simulink model "SM_Offshore_Windturbine"  (R2021a)
settings: Solver=ode4  StartTime=0.0  StopTime=par.sym.Ttot  FixedStep=par.sym.max_dt  MaxStep=par.sym.max_dt  RelTol=1e-3
model workspace: external: MATLAB File C:\Users\d053704\Desktop\MOST\Structure\CAD\CAD_DataFile.m (data not in the file)
undefined symbols (not defined in the file): par, smiData, X, Y, Z
libraries: sm_lib x50, simulink_extras x29, vrlib x18, nesl_utility x10, dspstat3 x9, sharedutil x5, eeGeneralControl x2
(part 3 of 4)

== system SM_Offshore_Windturbine/WIND TURBINE/BODIES MOTIONS/Simscape/Nacelle ==
  Nacelle : sm_lib/Body Elements/File Solid  ExtGeomFileName=Nacelle_Default_sldprt.STEP  UnitType=FromFile  ExtGeomFileUnits=m  StepReaderType=HEX  ExportConvexHullGeometry=off  InertiaType=Custom  Mass=smiData.Solid(5).mass  MassUnits=kg  CenterOfMass=smiData.Solid(5).CoM  CenterOfMassUnits=m  MomentsOfInertia=[eps eps eps]  MomentsOfInertiaUnits=kg*m^2  ProductsOfInertia=[0 0 0]  ProductsOfInertiaUnits=kg*m^2  BasedOnType=Density  Density=1000  DensityUnits=kg/m^3  DoExposeReferenceFrame=on  SerializedFrames=<Frames/>  GraphicType=FromGeometry  MarkerShape=Sphere  MarkerSize=10  GraphicVisPropType=SimpleVisualProperties  GraphicDiffuseColor=smiData.Solid(5).color  GraphicSpecularColor=[0.5 0.5 0.5 1.0]  GraphicAmbientColor=[0.15 0.15 0.15 1.0]  GraphicEmissiveColor=[0.0 0.0 0.0 1.0]  GraphicShininess=75  GraphicOpacity=smiData.Solid(5).opacity
  ReferenceFrame : sm_lib/Frames and Transforms/Reference Frame
  Transform1 : sm_lib/Frames and Transforms/Rigid Transform  TranslationMethod=Cartesian  TranslationStandardOffset=0  TranslationLengthUnit=m  TranslationStandardAxis=+Z  TranslationCartesianOffset=smiData.RigidTransform(9).translation  TranslationROffset=0  TranslationROffsetUnits=m  TranslationZOffset=0  TranslationZOffsetUnits=m  TranslationThetaOffset=0  TranslationThetaOffsetUnits=deg  RotationMethod=ArbitraryAxis  RotationAngleUnits=rad  RotationStandardAxis=+Z  RotationAngle=smiData.RigidTransform(9).angle  RotationArbitraryAxis=smiData.RigidTransform(9).axis  FollAlignAxisA=+X  BaseAlignAxisA=+Y  FollAlignAxisB=+Y  BaseAlignAxisB=+Z  RotationSequenceAxes=FollowerAxes  RotationSequence=XYX  RotationSequenceAngles=[0 0 0]  RotationSequenceAnglesUnits=deg  RotationMatrix=[1 0 0; 0 1 0; 0 0 1]
  Transform2 : sm_lib/Frames and Transforms/Rigid Transform  TranslationMethod=Cartesian  TranslationStandardOffset=0  TranslationLengthUnit=m  TranslationStandardAxis=+Z  TranslationCartesianOffset=smiData.RigidTransform(14).translation  TranslationROffset=0  TranslationROffsetUnits=m  TranslationZOffset=0  TranslationZOffsetUnits=m  TranslationThetaOffset=0  TranslationThetaOffsetUnits=deg  RotationMethod=ArbitraryAxis  RotationAngleUnits=rad  RotationStandardAxis=+Z  RotationAngle=smiData.RigidTransform(14).angle  RotationArbitraryAxis=smiData.RigidTransform(14).axis  FollAlignAxisA=+X  BaseAlignAxisA=+Y  FollAlignAxisB=+Y  BaseAlignAxisB=+Z  RotationSequenceAxes=FollowerAxes  RotationSequence=XYX  RotationSequenceAngles=[0 0 0]  RotationSequenceAnglesUnits=deg  RotationMatrix=[1 0 0; 0 1 0; 0 0 1]
  Transform4 : sm_lib/Frames and Transforms/Rigid Transform  TranslationMethod=Cartesian  TranslationStandardOffset=0  TranslationLengthUnit=m  TranslationStandardAxis=+Z  TranslationCartesianOffset=[0 0 0]  TranslationROffset=0  TranslationROffsetUnits=m  TranslationZOffset=0  TranslationZOffsetUnits=m  TranslationThetaOffset=0  TranslationThetaOffsetUnits=deg  RotationMethod=ArbitraryAxis  RotationAngleUnits=rad  RotationStandardAxis=+Z  RotationAngle=pi  RotationArbitraryAxis=[1 0 0]  FollAlignAxisA=+X  BaseAlignAxisA=+Y  FollAlignAxisB=+Y  BaseAlignAxisB=+Z  RotationSequenceAxes=FollowerAxes  RotationSequence=XYX  RotationSequenceAngles=[0 0 0]  RotationSequenceAnglesUnits=deg  RotationMatrix=[1 0 0; 0 1 0; 0 0 1]
  Tower : PMIOPort  Side=Left
  Rotor : PMIOPort  Port=2  Side=Right
  connections:
  Transform1/LConn1 -- ReferenceFrame/RConn1 -- Nacelle/RConn1 -- Transform2/LConn1
  Transform4/RConn1 -- Rotor/RConn1
  Transform2/RConn1 -- Tower/RConn1
  Transform1/RConn1 -- Transform4/LConn1

== system SM_Offshore_Windturbine/WIND TURBINE/BODIES MOTIONS/Simscape/Rotor ==
  ReferenceFrame : sm_lib/Frames and Transforms/Reference Frame
  Rotor : sm_lib/Body Elements/File Solid  ExtGeomFileName=Rotor_Default_sldprt.STEP  UnitType=FromFile  ExtGeomFileUnits=m  StepReaderType=HEX  ExportConvexHullGeometry=off  InertiaType=Custom  Mass=67550  MassUnits=kg  CenterOfMass=smiData.Solid(3).CoM  CenterOfMassUnits=m  MomentsOfInertia=[par.WT.prop.Idt 0 0]  MomentsOfInertiaUnits=kg*m^2  ProductsOfInertia=[0 0 0]  ProductsOfInertiaUnits=kg*m^2  BasedOnType=Density  Density=1000  DensityUnits=kg/m^3  DoExposeReferenceFrame=on  SerializedFrames=<Frames/>  GraphicType=FromGeometry  MarkerShape=Sphere  MarkerSize=10  GraphicVisPropType=SimpleVisualProperties  GraphicDiffuseColor=smiData.Solid(3).color  GraphicSpecularColor=[0.5 0.5 0.5 1.0]  GraphicAmbientColor=[0.15 0.15 0.15 1.0]  GraphicEmissiveColor=[0.0 0.0 0.0 1.0]  GraphicShininess=75  GraphicOpacity=smiData.Solid(3).opacity
  Transform : sm_lib/Frames and Transforms/Rigid Transform  TranslationMethod=Cartesian  TranslationStandardOffset=0  TranslationLengthUnit=m  TranslationStandardAxis=+Z  TranslationCartesianOffset=smiData.RigidTransform(1).translation  TranslationROffset=0  TranslationROffsetUnits=m  TranslationZOffset=0  TranslationZOffsetUnits=m  TranslationThetaOffset=0  TranslationThetaOffsetUnits=deg  RotationMethod=ArbitraryAxis  RotationAngleUnits=rad  RotationStandardAxis=+Z  RotationAngle=smiData.RigidTransform(1).angle  RotationArbitraryAxis=smiData.RigidTransform(1).axis  FollAlignAxisA=+X  BaseAlignAxisA=+Y  FollAlignAxisB=+Y  BaseAlignAxisB=+Z  RotationSequenceAxes=FollowerAxes  RotationSequence=XYX  RotationSequenceAngles=[0 0 0]  RotationSequenceAnglesUnits=deg  RotationMatrix=[1 0 0; 0 1 0; 0 0 1]
  Transform1 : sm_lib/Frames and Transforms/Rigid Transform  TranslationMethod=Cartesian  TranslationStandardOffset=0  TranslationLengthUnit=m  TranslationStandardAxis=+Z  TranslationCartesianOffset=smiData.RigidTransform(3).translation  TranslationROffset=0  TranslationROffsetUnits=m  TranslationZOffset=0  TranslationZOffsetUnits=m  TranslationThetaOffset=0  TranslationThetaOffsetUnits=deg  RotationMethod=ArbitraryAxis  RotationAngleUnits=rad  RotationStandardAxis=+Z  RotationAngle=smiData.RigidTransform(3).angle  RotationArbitraryAxis=smiData.RigidTransform(3).axis  FollAlignAxisA=+X  BaseAlignAxisA=+Y  FollAlignAxisB=+Y  BaseAlignAxisB=+Z  RotationSequenceAxes=FollowerAxes  RotationSequence=XYX  RotationSequenceAngles=[0 0 0]  RotationSequenceAnglesUnits=deg  RotationMatrix=[1 0 0; 0 1 0; 0 0 1]
  Transform2 : sm_lib/Frames and Transforms/Rigid Transform  TranslationMethod=Cartesian  TranslationStandardOffset=0  TranslationLengthUnit=m  TranslationStandardAxis=+Z  TranslationCartesianOffset=smiData.RigidTransform(5).translation  TranslationROffset=0  TranslationROffsetUnits=m  TranslationZOffset=0  TranslationZOffsetUnits=m  TranslationThetaOffset=0  TranslationThetaOffsetUnits=deg  RotationMethod=ArbitraryAxis  RotationAngleUnits=rad  RotationStandardAxis=+Z  RotationAngle=smiData.RigidTransform(5).angle  RotationArbitraryAxis=smiData.RigidTransform(5).axis  FollAlignAxisA=+X  BaseAlignAxisA=+Y  FollAlignAxisB=+Y  BaseAlignAxisB=+Z  RotationSequenceAxes=FollowerAxes  RotationSequence=XYX  RotationSequenceAngles=[0 0 0]  RotationSequenceAnglesUnits=deg  RotationMatrix=[1 0 0; 0 1 0; 0 0 1]
  Transform3 : sm_lib/Frames and Transforms/Rigid Transform  TranslationMethod=Cartesian  TranslationStandardOffset=0  TranslationLengthUnit=m  TranslationStandardAxis=+Z  TranslationCartesianOffset=smiData.RigidTransform(10).translation  TranslationROffset=0  TranslationROffsetUnits=m  TranslationZOffset=0  TranslationZOffsetUnits=m  TranslationThetaOffset=0  TranslationThetaOffsetUnits=deg  RotationMethod=ArbitraryAxis  RotationAngleUnits=rad  RotationStandardAxis=+Z  RotationAngle=smiData.RigidTransform(10).angle  RotationArbitraryAxis=smiData.RigidTransform(10).axis  FollAlignAxisA=+X  BaseAlignAxisA=+Y  FollAlignAxisB=+Y  BaseAlignAxisB=+Z  RotationSequenceAxes=FollowerAxes  RotationSequence=XYX  RotationSequenceAngles=[0 0 0]  RotationSequenceAnglesUnits=deg  RotationMatrix=[1 0 0; 0 1 0; 0 0 1]
  Transform4 : sm_lib/Frames and Transforms/Rigid Transform  TranslationMethod=Cartesian  TranslationStandardOffset=0  TranslationLengthUnit=m  TranslationStandardAxis=+Z  TranslationCartesianOffset=[0 0 0]  TranslationROffset=0  TranslationROffsetUnits=m  TranslationZOffset=0  TranslationZOffsetUnits=m  TranslationThetaOffset=0  TranslationThetaOffsetUnits=deg  RotationMethod=ArbitraryAxis  RotationAngleUnits=rad  RotationStandardAxis=+Z  RotationAngle=pi  RotationArbitraryAxis=[1 0 0]  FollAlignAxisA=+X  BaseAlignAxisA=+Y  FollAlignAxisB=+Y  BaseAlignAxisB=+Z  RotationSequenceAxes=FollowerAxes  RotationSequence=XYX  RotationSequenceAngles=[0 0 0]  RotationSequenceAnglesUnits=deg  RotationMatrix=[1 0 0; 0 1 0; 0 0 1]
  Nacelle : PMIOPort  Side=Left
  Blade3 : PMIOPort  Port=2  Side=Right
  Blade2 : PMIOPort  Port=3  Side=Right
  Blade1 : PMIOPort  Port=4  Side=Right
  connections:
  ReferenceFrame/RConn1 -- Transform2/LConn1 -- Transform3/LConn1 -- Transform/LConn1 -- Transform1/LConn1 -- Rotor/RConn1
  Transform/RConn1 -- Blade1/RConn1
  Transform1/RConn1 -- Blade2/RConn1
  Transform2/RConn1 -- Blade3/RConn1
  Transform3/RConn1 -- Transform4/LConn1
  Transform4/RConn1 -- Nacelle/RConn1

== system SM_Offshore_Windturbine/WIND TURBINE/BODIES MOTIONS/Simscape/Spar OC3 ==
  ReferenceFrame : sm_lib/Frames and Transforms/Reference Frame
  Substructure : sm_lib/Body Elements/File Solid  ExtGeomFileName=oc3.IGS  UnitType=FromFile  ExtGeomFileUnits=m  StepReaderType=HEX  ExportConvexHullGeometry=off  InertiaType=Custom  Mass=smiData.Solid(2).mass  MassUnits=kg  CenterOfMass=smiData.Solid(2).CoM  CenterOfMassUnits=m  MomentsOfInertia=[eps eps eps]  MomentsOfInertiaUnits=kg*m^2  ProductsOfInertia=[0 0 0]  ProductsOfInertiaUnits=kg*m^2  BasedOnType=Density  Density=1000  DensityUnits=kg/m^3  DoExposeReferenceFrame=on  SerializedFrames=<Frames/>  GraphicType=FromGeometry  MarkerShape=Sphere  MarkerSize=10  GraphicVisPropType=SimpleVisualProperties  GraphicDiffuseColor=[1.0 0.8627451 0.11764706]  GraphicSpecularColor=[0.5 0.5 0.5 1.0]  GraphicAmbientColor=[0.15 0.15 0.15 1.0]  GraphicEmissiveColor=[0.0 0.0 0.0 1.0]  GraphicShininess=75  GraphicOpacity=smiData.Solid(2).opacity
  Transform : sm_lib/Frames and Transforms/Rigid Transform  TranslationMethod=Cartesian  TranslationStandardOffset=0  TranslationLengthUnit=m  TranslationStandardAxis=+Z  TranslationCartesianOffset=smiData.RigidTransform(16).translation  TranslationROffset=0  TranslationROffsetUnits=m  TranslationZOffset=0  TranslationZOffsetUnits=m  TranslationThetaOffset=0  TranslationThetaOffsetUnits=deg  RotationMethod=ArbitraryAxis  RotationAngleUnits=rad  RotationStandardAxis=+Z  RotationAngle=smiData.RigidTransform(16).angle  RotationArbitraryAxis=smiData.RigidTransform(16).axis  FollAlignAxisA=+X  BaseAlignAxisA=+Y  FollAlignAxisB=+Y  BaseAlignAxisB=+Z  RotationSequenceAxes=FollowerAxes  RotationSequence=XYX  RotationSequenceAngles=[0 0 0]  RotationSequenceAnglesUnits=deg  RotationMatrix=[1 0 0; 0 1 0; 0 0 1]
  Transform1 : sm_lib/Frames and Transforms/Rigid Transform  TranslationMethod=Cartesian  TranslationStandardOffset=0  TranslationLengthUnit=m  TranslationStandardAxis=+Z  TranslationCartesianOffset=[0 0 0]  TranslationROffset=0  TranslationROffsetUnits=m  TranslationZOffset=0  TranslationZOffsetUnits=m  TranslationThetaOffset=0  TranslationThetaOffsetUnits=deg  RotationMethod=ArbitraryAxis  RotationAngleUnits=rad  RotationStandardAxis=+Z  RotationAngle=pi  RotationArbitraryAxis=[0 1 0]  FollAlignAxisA=+X  BaseAlignAxisA=+Y  FollAlignAxisB=+Y  BaseAlignAxisB=+Z  RotationSequenceAxes=FollowerAxes  RotationSequence=XYX  RotationSequenceAngles=[0 0 0]  RotationSequenceAnglesUnits=deg  RotationMatrix=[1 0 0; 0 1 0; 0 0 1]
  Transform2 : sm_lib/Frames and Transforms/Rigid Transform  TranslationMethod=Cartesian  TranslationStandardOffset=0  TranslationLengthUnit=m  TranslationStandardAxis=+Z  TranslationCartesianOffset=[0 0 0]  TranslationROffset=0  TranslationROffsetUnits=m  TranslationZOffset=0  TranslationZOffsetUnits=m  TranslationThetaOffset=0  TranslationThetaOffsetUnits=deg  RotationMethod=ArbitraryAxis  RotationAngleUnits=rad  RotationStandardAxis=+Z  RotationAngle=pi/2  RotationArbitraryAxis=[0 0 1]  FollAlignAxisA=+X  BaseAlignAxisA=+Y  FollAlignAxisB=+Y  BaseAlignAxisB=+Z  RotationSequenceAxes=FollowerAxes  RotationSequence=XYX  RotationSequenceAngles=[0 0 0]  RotationSequenceAnglesUnits=deg  RotationMatrix=[1 0 0; 0 1 0; 0 0 1]
  Transform3 : sm_lib/Frames and Transforms/Rigid Transform  TranslationMethod=Cartesian  TranslationStandardOffset=0  TranslationLengthUnit=m  TranslationStandardAxis=+Z  TranslationCartesianOffset=[0 -2 0]  TranslationROffset=0  TranslationROffsetUnits=m  TranslationZOffset=0  TranslationZOffsetUnits=m  TranslationThetaOffset=0  TranslationThetaOffsetUnits=deg  RotationMethod=ArbitraryAxis  RotationAngleUnits=rad  RotationStandardAxis=+Z  RotationAngle=0  RotationArbitraryAxis=[0 0 0]  FollAlignAxisA=+X  BaseAlignAxisA=+Y  FollAlignAxisB=+Y  BaseAlignAxisB=+Z  RotationSequenceAxes=FollowerAxes  RotationSequence=XYX  RotationSequenceAngles=[0 0 0]  RotationSequenceAnglesUnits=deg  RotationMatrix=[1 0 0; 0 1 0; 0 0 1]
  Transform4 : sm_lib/Frames and Transforms/Rigid Transform  TranslationMethod=Cartesian  TranslationStandardOffset=0  TranslationLengthUnit=m  TranslationStandardAxis=+Z  TranslationCartesianOffset=[0 3.22 0]  TranslationROffset=0  TranslationROffsetUnits=m  TranslationZOffset=0  TranslationZOffsetUnits=m  TranslationThetaOffset=0  TranslationThetaOffsetUnits=deg  RotationMethod=ArbitraryAxis  RotationAngleUnits=rad  RotationStandardAxis=+Z  RotationAngle=0  RotationArbitraryAxis=[0 0 0]  FollAlignAxisA=+X  BaseAlignAxisA=+Y  FollAlignAxisB=+Y  BaseAlignAxisB=+Z  RotationSequenceAxes=FollowerAxes  RotationSequence=XYX  RotationSequenceAngles=[0 0 0]  RotationSequenceAnglesUnits=deg  RotationMatrix=[1 0 0; 0 1 0; 0 0 1]
  Transform5 : sm_lib/Frames and Transforms/Rigid Transform  TranslationMethod=Cartesian  TranslationStandardOffset=0  TranslationLengthUnit=m  TranslationStandardAxis=+Z  TranslationCartesianOffset=[0 0 0]  TranslationROffset=0  TranslationROffsetUnits=m  TranslationZOffset=0  TranslationZOffsetUnits=m  TranslationThetaOffset=0  TranslationThetaOffsetUnits=deg  RotationMethod=ArbitraryAxis  RotationAngleUnits=rad  RotationStandardAxis=+Z  RotationAngle=pi/2  RotationArbitraryAxis=[0 0 1]  FollAlignAxisA=+X  BaseAlignAxisA=+Y  FollAlignAxisB=+Y  BaseAlignAxisB=+Z  RotationSequenceAxes=FollowerAxes  RotationSequence=XYX  RotationSequenceAngles=[0 0 0]  RotationSequenceAnglesUnits=deg  RotationMatrix=[1 0 0; 0 1 0; 0 0 1]
  Transform6 : sm_lib/Frames and Transforms/Rigid Transform  TranslationMethod=Cartesian  TranslationStandardOffset=0  TranslationLengthUnit=m  TranslationStandardAxis=+Z  TranslationCartesianOffset=[0 0 0]  TranslationROffset=0  TranslationROffsetUnits=m  TranslationZOffset=0  TranslationZOffsetUnits=m  TranslationThetaOffset=0  TranslationThetaOffsetUnits=deg  RotationMethod=ArbitraryAxis  RotationAngleUnits=rad  RotationStandardAxis=+Z  RotationAngle=pi  RotationArbitraryAxis=[0 1 0]  FollAlignAxisA=+X  BaseAlignAxisA=+Y  FollAlignAxisB=+Y  BaseAlignAxisB=+Z  RotationSequenceAxes=FollowerAxes  RotationSequence=XYX  RotationSequenceAngles=[0 0 0]  RotationSequenceAnglesUnits=deg  RotationMatrix=[1 0 0; 0 1 0; 0 0 1]
  Transform7 : sm_lib/Frames and Transforms/Rigid Transform  TranslationMethod=Cartesian  TranslationStandardOffset=0  TranslationLengthUnit=m  TranslationStandardAxis=+Z  TranslationCartesianOffset=[0 0 0]  TranslationROffset=0  TranslationROffsetUnits=m  TranslationZOffset=0  TranslationZOffsetUnits=m  TranslationThetaOffset=0  TranslationThetaOffsetUnits=deg  RotationMethod=ArbitraryAxis  RotationAngleUnits=rad  RotationStandardAxis=+Z  RotationAngle=smiData.RigidTransform(16).angle  RotationArbitraryAxis=smiData.RigidTransform(16).axis  FollAlignAxisA=+X  BaseAlignAxisA=+Y  FollAlignAxisB=+Y  BaseAlignAxisB=+Z  RotationSequenceAxes=FollowerAxes  RotationSequence=XYX  RotationSequenceAngles=[0 0 0]  RotationSequenceAnglesUnits=deg  RotationMatrix=[1 0 0; 0 1 0; 0 0 1]
  tower : PMIOPort  Side=Right
  F1 : PMIOPort  Port=2  Side=Left
  connections:
  Transform/LConn1 -- Transform3/LConn1 -- ReferenceFrame/RConn1 -- Substructure/RConn1
  Transform2/RConn1 -- tower/RConn1
  Transform/RConn1 -- Transform4/LConn1
  Transform4/RConn1 -- Transform1/LConn1
  Transform1/RConn1 -- Transform2/LConn1
  Transform3/RConn1 -- Transform7/LConn1
  Transform5/RConn1 -- F1/RConn1
  Transform6/RConn1 -- Transform5/LConn1
  Transform7/RConn1 -- Transform6/LConn1

== system SM_Offshore_Windturbine/WIND TURBINE/BODIES MOTIONS/Simscape/Tower ==
  ReferenceFrame : sm_lib/Frames and Transforms/Reference Frame
  Tower : sm_lib/Body Elements/File Solid  ExtGeomFileName=Tower_Default_sldprt.STEP  UnitType=FromFile  ExtGeomFileUnits=m  StepReaderType=HEX  ExportConvexHullGeometry=off  InertiaType=Custom  Mass=297150  MassUnits=kg  CenterOfMass=smiData.Solid(4).CoM  CenterOfMassUnits=m  MomentsOfInertia=[eps eps eps]  MomentsOfInertiaUnits=kg*m^2  ProductsOfInertia=[0 0 0]  ProductsOfInertiaUnits=kg*m^2  BasedOnType=Density  Density=1000  DensityUnits=kg/m^3  DoExposeReferenceFrame=on  SerializedFrames=<Frames/>  GraphicType=FromGeometry  MarkerShape=Sphere  MarkerSize=10  GraphicVisPropType=SimpleVisualProperties  GraphicDiffuseColor=smiData.Solid(4).color  GraphicSpecularColor=[0.5 0.5 0.5 1.0]  GraphicAmbientColor=[0.15 0.15 0.15 1.0]  GraphicEmissiveColor=[0.0 0.0 0.0 1.0]  GraphicShininess=75  GraphicOpacity=smiData.Solid(4).opacity
  Transform1 : sm_lib/Frames and Transforms/Rigid Transform  TranslationMethod=Cartesian  TranslationStandardOffset=0  TranslationLengthUnit=m  TranslationStandardAxis=+Z  TranslationCartesianOffset=smiData.RigidTransform(13).translation  TranslationROffset=0  TranslationROffsetUnits=m  TranslationZOffset=0  TranslationZOffsetUnits=m  TranslationThetaOffset=0  TranslationThetaOffsetUnits=deg  RotationMethod=ArbitraryAxis  RotationAngleUnits=rad  RotationStandardAxis=+Z  RotationAngle=smiData.RigidTransform(13).angle  RotationArbitraryAxis=smiData.RigidTransform(13).axis  FollAlignAxisA=+X  BaseAlignAxisA=+Y  FollAlignAxisB=+Y  BaseAlignAxisB=+Z  RotationSequenceAxes=FollowerAxes  RotationSequence=XYX  RotationSequenceAngles=[0 0 0]  RotationSequenceAnglesUnits=deg  RotationMatrix=[1 0 0; 0 1 0; 0 0 1]
  Transform2 : sm_lib/Frames and Transforms/Rigid Transform  TranslationMethod=Cartesian  TranslationStandardOffset=0  TranslationLengthUnit=m  TranslationStandardAxis=+Z  TranslationCartesianOffset=smiData.RigidTransform(15).translation  TranslationROffset=0  TranslationROffsetUnits=m  TranslationZOffset=0  TranslationZOffsetUnits=m  TranslationThetaOffset=0  TranslationThetaOffsetUnits=deg  RotationMethod=ArbitraryAxis  RotationAngleUnits=rad  RotationStandardAxis=+Z  RotationAngle=smiData.RigidTransform(15).angle  RotationArbitraryAxis=smiData.RigidTransform(15).axis  FollAlignAxisA=+X  BaseAlignAxisA=+Y  FollAlignAxisB=+Y  BaseAlignAxisB=+Z  RotationSequenceAxes=FollowerAxes  RotationSequence=XYX  RotationSequenceAngles=[0 0 0]  RotationSequenceAnglesUnits=deg  RotationMatrix=[1 0 0; 0 1 0; 0 0 1]
  Transform3 : sm_lib/Frames and Transforms/Rigid Transform  TranslationMethod=Cartesian  TranslationStandardOffset=0  TranslationLengthUnit=m  TranslationStandardAxis=+Z  TranslationCartesianOffset=[0 0 0]  TranslationROffset=0  TranslationROffsetUnits=m  TranslationZOffset=0  TranslationZOffsetUnits=m  TranslationThetaOffset=0  TranslationThetaOffsetUnits=deg  RotationMethod=ArbitraryAxis  RotationAngleUnits=rad  RotationStandardAxis=+Z  RotationAngle=pi  RotationArbitraryAxis=[0 1 0]  FollAlignAxisA=+X  BaseAlignAxisA=+Y  FollAlignAxisB=+Y  BaseAlignAxisB=+Z  RotationSequenceAxes=FollowerAxes  RotationSequence=XYX  RotationSequenceAngles=[0 0 0]  RotationSequenceAnglesUnits=deg  RotationMatrix=[1 0 0; 0 1 0; 0 0 1]
  Transform4 : sm_lib/Frames and Transforms/Rigid Transform  TranslationMethod=Cartesian  TranslationStandardOffset=0  TranslationLengthUnit=m  TranslationStandardAxis=+Z  TranslationCartesianOffset=[0 3.22 0]  TranslationROffset=0  TranslationROffsetUnits=m  TranslationZOffset=0  TranslationZOffsetUnits=m  TranslationThetaOffset=0  TranslationThetaOffsetUnits=deg  RotationMethod=ArbitraryAxis  RotationAngleUnits=rad  RotationStandardAxis=+Z  RotationAngle=0  RotationArbitraryAxis=[0 0 0]  FollAlignAxisA=+X  BaseAlignAxisA=+Y  FollAlignAxisB=+Y  BaseAlignAxisB=+Z  RotationSequenceAxes=FollowerAxes  RotationSequence=XYX  RotationSequenceAngles=[0 0 0]  RotationSequenceAnglesUnits=deg  RotationMatrix=[1 0 0; 0 1 0; 0 0 1]
  Transform5 : sm_lib/Frames and Transforms/Rigid Transform  TranslationMethod=Cartesian  TranslationStandardOffset=0  TranslationLengthUnit=m  TranslationStandardAxis=+Z  TranslationCartesianOffset=[0 0 0]  TranslationROffset=0  TranslationROffsetUnits=m  TranslationZOffset=0  TranslationZOffsetUnits=m  TranslationThetaOffset=0  TranslationThetaOffsetUnits=deg  RotationMethod=ArbitraryAxis  RotationAngleUnits=rad  RotationStandardAxis=+Z  RotationAngle=pi/2  RotationArbitraryAxis=[0 0 1]  FollAlignAxisA=+X  BaseAlignAxisA=+Y  FollAlignAxisB=+Y  BaseAlignAxisB=+Z  RotationSequenceAxes=FollowerAxes  RotationSequence=XYX  RotationSequenceAngles=[0 0 0]  RotationSequenceAnglesUnits=deg  RotationMatrix=[1 0 0; 0 1 0; 0 0 1]
  Base : PMIOPort  Side=Left
  Nacelle : PMIOPort  Port=2  Side=Right
  connections:
  Transform1/LConn1 -- ReferenceFrame/RConn1 -- Tower/RConn1 -- Transform2/LConn1
  Transform1/RConn1 -- Nacelle/RConn1
  Transform4/RConn1 -- Transform3/LConn1
  Transform4/LConn1 -- Transform2/RConn1
  Transform5/RConn1 -- Base/RConn1
  Transform3/RConn1 -- Transform5/LConn1

== system SM_Offshore_Windturbine/WIND TURBINE/CONTROL SYSTEM/TORQUE CONTROL/Constant Power Law ==
  BlPtch>0 : Inport
  Action Port : ActionPort  ActionPortLabel=if(u1 > u2)
  Constant : Constant  Value=par.WT.ctrl.PTO.Pwnom
  Product : Product
  Reciprocal : Product  Inputs=/
  Saturation : Saturate  UpperLimit=par.WT.ctrl.PTO.Tnom*1.1  LowerLimit=0
  " " : Outport  VectorParamsAs1DForOutWhenUnconnected=off
  wires:
  Saturation/1 -> " "/1
  BlPtch>0/1 -> Reciprocal/1
  Reciprocal/1 -> Product/2
  Constant/1 -> Product/1
  Product/1 -> Saturation/1

== system SM_Offshore_Windturbine/WIND TURBINE/CONTROL SYSTEM/TORQUE CONTROL/Constant Torque Law ==
  BlPtch=0 : Inport
  Action Port : ActionPort  ActionPortLabel=else
  " " : Outport  VectorParamsAs1DForOutWhenUnconnected=off
  wires:
  BlPtch=0/1 -> " "/1

== system SM_Offshore_Windturbine/WIND TURBINE/ROTOR LOADS/Aerodynamic Loads/Blade 1 ==
  Azimuth : Inport
  Omega : Inport  Port=2
  blade pitch : Inport  Port=3
  6 DOF : Inport  Port=4
  Time : Inport  Port=5
  BEM : Subsystem  TreatAsAtomicUnit=on
  Gain : Gain  Gain=1/3
  Post_processing : MATLAB Function  TreatAsAtomicUnit=on
  AIF : Outport  VectorParamsAs1DForOutWhenUnconnected=off
  TIF : Outport  Port=2  VectorParamsAs1DForOutWhenUnconnected=off
  Azimuth1 : Outport  Port=3  VectorParamsAs1DForOutWhenUnconnected=off
  Cn : Outport  Port=4  VectorParamsAs1DForOutWhenUnconnected=off
  Ct : Outport  Port=5  VectorParamsAs1DForOutWhenUnconnected=off
  Vx : Outport  Port=6  VectorParamsAs1DForOutWhenUnconnected=off
  Vy : Outport  Port=7  VectorParamsAs1DForOutWhenUnconnected=off
  V0 : Outport  Port=8  VectorParamsAs1DForOutWhenUnconnected=off
  wires:
  Omega/1 -> BEM/2(Rotor speed)
  Azimuth/1 -> BEM/1(Azimuth)
  6 DOF/1 -> BEM/4(6 DOF)
  blade pitch/1 -> BEM/3(Blade pitch)
  Time/1 -> BEM/5(Time)
  BEM/3(TIF) -> Post_processing/2("TIF ")
  Post_processing/1(AIF) -> AIF/1
  Post_processing/2(TIF) -> TIF/1
  BEM/1(Azimuth 1) -> Azimuth1/1
  BEM/2(AIF) -> Post_processing/1("AIF ")
  BEM/4(Cn) -> Cn/1
  BEM/5(Ct) -> Ct/1
  BEM/6(Vx) -> Vx/1
  BEM/7(Vy) -> Vy/1
  BEM/8(V0) -> Gain/1
  Gain/1 -> V0/1

== system SM_Offshore_Windturbine/WIND TURBINE/ROTOR LOADS/Aerodynamic Loads/Blade 2 ==
  Azimuth : Inport
  Omega : Inport  Port=2
  blade pitch : Inport  Port=3
  6 DOF : Inport  Port=4
  Time : Inport  Port=5
  BEM : Subsystem  TreatAsAtomicUnit=on
  Gain : Gain  Gain=1/3
  Post_processing : MATLAB Function  TreatAsAtomicUnit=on
  AIF : Outport  VectorParamsAs1DForOutWhenUnconnected=off
  TIF : Outport  Port=2  VectorParamsAs1DForOutWhenUnconnected=off
  Azimuth2 : Outport  Port=3  VectorParamsAs1DForOutWhenUnconnected=off
  Cn : Outport  Port=4  VectorParamsAs1DForOutWhenUnconnected=off
  Ct : Outport  Port=5  VectorParamsAs1DForOutWhenUnconnected=off
  Vx : Outport  Port=6  VectorParamsAs1DForOutWhenUnconnected=off
  Vy : Outport  Port=7  VectorParamsAs1DForOutWhenUnconnected=off
  V0 : Outport  Port=8  VectorParamsAs1DForOutWhenUnconnected=off
  wires:
  Omega/1 -> BEM/2(Rotor speed)
  Azimuth/1 -> BEM/1(Azimuth)
  6 DOF/1 -> BEM/4(6 DOF)
  blade pitch/1 -> BEM/3(Blade pitch)
  Time/1 -> BEM/5(Time)
  BEM/3(TIF) -> Post_processing/2("TIF ")
  Post_processing/1(AIF) -> AIF/1
  Post_processing/2(TIF) -> TIF/1
  BEM/1(Azimuth 2) -> Azimuth2/1
  BEM/2(AIF) -> Post_processing/1("AIF ")
  BEM/4(Cn) -> Cn/1
  BEM/5(Ct) -> Ct/1
  BEM/6(Vx) -> Vx/1
  BEM/7(Vy) -> Vy/1
  BEM/8(V0) -> Gain/1
  Gain/1 -> V0/1

== system SM_Offshore_Windturbine/WIND TURBINE/ROTOR LOADS/Aerodynamic Loads/Blade 3 ==
  Azimuth : Inport
  Omega : Inport  Port=2
  blade pitch : Inport  Port=3
  6 DOF : Inport  Port=4
  Time : Inport  Port=5
  BEM : Subsystem  TreatAsAtomicUnit=on
  Gain : Gain  Gain=1/3
  Post_processing : MATLAB Function  TreatAsAtomicUnit=on
  AIF : Outport  VectorParamsAs1DForOutWhenUnconnected=off
  TIF : Outport  Port=2  VectorParamsAs1DForOutWhenUnconnected=off
  Azimuth3 : Outport  Port=3  VectorParamsAs1DForOutWhenUnconnected=off
  Cn : Outport  Port=4  VectorParamsAs1DForOutWhenUnconnected=off
  Ct : Outport  Port=5  VectorParamsAs1DForOutWhenUnconnected=off
  Vx : Outport  Port=6  VectorParamsAs1DForOutWhenUnconnected=off
  Vy : Outport  Port=7  VectorParamsAs1DForOutWhenUnconnected=off
  V0 : Outport  Port=8  VectorParamsAs1DForOutWhenUnconnected=off
  wires:
  BEM/7(Vy) -> Vy/1
  BEM/6(Vx) -> Vx/1
  BEM/5(Ct) -> Ct/1
  BEM/4(Cn) -> Cn/1
  BEM/2(AIF) -> Post_processing/1("AIF ")
  BEM/1(Azimuth 3) -> Azimuth3/1
  Post_processing/2(TIF) -> TIF/1
  Post_processing/1(AIF) -> AIF/1
  BEM/3(TIF) -> Post_processing/2("TIF ")
  Time/1 -> BEM/5(Time)
  blade pitch/1 -> BEM/3(Blade pitch)
  6 DOF/1 -> BEM/4(6 DOF)
  Azimuth/1 -> BEM/1(Azimuth)
  Omega/1 -> BEM/2(Rotor speed)
  BEM/8(V0) -> Gain/1
  Gain/1 -> V0/1

== system SM_Offshore_Windturbine/WIND TURBINE/ROTOR LOADS/TowerBaseLoads/3D rotation matrix ==
  hull_rotation : Inport
  Constant : Constant
  Create 3x3 Matrix : sharedutil/Create 3x3 Matrix  aMode=aMode
      settings: SourceProductBaseCode=AE,PW,DR,MT,UV,VE
  Fcn1 : Fcn  Expr=u(2)*u(7) + u(3)*u(1)*(u(8)-1)
  Fcn11 : Fcn  Expr=u(4)*u(8) + u(5) + u(6)
  Fcn2 : Fcn  Expr=-u(2)*u(7) + u(1)*u(3)*(u(8)-1)
  Fcn3 : Fcn  Expr=u(5)*u(8) + u(4) + u(6)
  Fcn4 : Fcn  Expr=-u(1)*u(7) + u(3)*u(2)*(u(8)-1)
  Fcn5 : Fcn  Expr=u(1)*u(7) + u(3)*u(2)*(u(8)-1)
  Fcn7 : Fcn  Expr=u(6)*u(8) + u(4) + u(5)
  Fcn8 : Fcn  Expr=u(3)*u(7) + u(1)*u(2)*(u(8)-1)
  Fcn9 : Fcn  Expr=-u(3)*u(7) + u(1)*u(2)*(u(8)-1)
  If : If  IfExpression=u1 == 0
  If Action Subsystem : Subsystem  TreatAsAtomicUnit=on
  If Action Subsystem1 : Subsystem  TreatAsAtomicUnit=on
  Merge : Merge
  Mux : Mux  Inputs=8
  Sqrt : Sqrt  SaturateOnIntegerOverflow=on
  Sum : Sum  Inputs=+++|
  Sum1 : Sum  Inputs=++|
  TETA1 : Math  Operator=square  SignedPower=on  SaturateOnIntegerOverflow=on
  TETA2 : Math  Operator=square  SignedPower=on  SaturateOnIntegerOverflow=on
  TETA3 : Math  Operator=square  SignedPower=on  SaturateOnIntegerOverflow=on
  teta1 : Selector  InputPortWidth=3  IndexOptions=Index vector (dialog)  Indices=1  OutputSizes=1
  teta2 : Selector  InputPortWidth=3  IndexOptions=Index vector (dialog)  Indices=2  OutputSizes=1
  teta3 : Selector  InputPortWidth=3  IndexOptions=Index vector (dialog)  Indices=3  OutputSizes=1
  R(rx,ry,rz) : Outport  VectorParamsAs1DForOutWhenUnconnected=off
  wires:
  hull_rotation/1 -> teta1/1, teta3/1, teta2/1
  teta1/1 -> Mux/1, TETA1/1
  teta2/1 -> Mux/2, TETA2/1
  teta3/1 -> Mux/3, TETA3/1
  TETA2/1 -> Mux/5, Sum/2
  TETA1/1 -> Mux/4, Sum/1
  TETA3/1 -> Mux/6, Sum/3
  Sum/1 -> Mux/7, Sum1/1, If Action Subsystem1/1(TETA), If/1  "TETA"
  Sum1/1 -> Sqrt/1
  Sqrt/1 -> If Action Subsystem1/2(rad), Mux/8  "rad"
  Fcn4/1 -> Create 3x3 Matrix/6
  Fcn3/1 -> Create 3x3 Matrix/5
  Fcn8/1 -> Create 3x3 Matrix/4
  Fcn2/1 -> Create 3x3 Matrix/7
  Fcn1/1 -> Create 3x3 Matrix/3
  Fcn7/1 -> Create 3x3 Matrix/9
  Fcn11/1 -> Create 3x3 Matrix/1
  Fcn5/1 -> Create 3x3 Matrix/8
  Fcn9/1 -> Create 3x3 Matrix/2
  Mux/1 -> Fcn3/1, Fcn4/1, Fcn2/1, Fcn5/1, Fcn7/1, Fcn8/1, Fcn1/1, Fcn9/1, Fcn11/1
  Constant/1 -> Sum1/2
  If/2 -> If Action Subsystem1/Action
  If Action Subsystem/1(R) -> Merge/2
  Merge/1 -> R(rx,ry,rz)/1
  If/1 -> If Action Subsystem/Action
  If Action Subsystem1/1(R) -> Merge/1
  Create 3x3 Matrix/1 -> If Action Subsystem1/3(T)

== system SM_Offshore_Windturbine/HULL/Viscous loads/Subsystem1/3D rotation matrix/If Action Subsystem ==
  Action Port : ActionPort  ActionPortLabel=if(u1 == 0)
  Constant : Constant  Value=[1 0 0; 0 1 0; 0 0 1]
  R : Outport  VectorParamsAs1DForOutWhenUnconnected=off
  wires:
  Constant/1 -> R/1

== system SM_Offshore_Windturbine/HULL/Viscous loads/Subsystem1/3D rotation matrix/If Action Subsystem1 ==
  TETA : Inport
  rad : Inport  Port=2
  T : Inport  Port=3
  Action Port : ActionPort  ActionPortLabel=else
  Divide : Product  Inputs=//*
  R : Outport  VectorParamsAs1DForOutWhenUnconnected=off
  wires:
  T/1 -> Divide/3
  TETA/1 -> Divide/1
  rad/1 -> Divide/2
  Divide/1 -> R/1

== system SM_Offshore_Windturbine/HULL/Viscous loads/Subsystem1/Wave velocities/Subsystem ==
  Hull rot spd : Inport
  Zrot1 : Inport  Port=2
  Zplat : Inport  Port=3
  VxVec : Inport  Port=4
  VyVec : Inport  Port=5
  Constant1 : Constant  Value=par.wave.velocities.Z
  Cross Product : vrlib/Utilities/Cross Product
  Interpolation Using Prelookup : Interpolation_n-D  NumberOfTableDimensions=1  TableSource=Input port  InternalRulePriority=Speed
      settings: InputPortMap=u0,u1,p2
  Interpolation Using Prelookup1 : Interpolation_n-D  NumberOfTableDimensions=1  TableSource=Input port  InternalRulePriority=Speed
      settings: InputPortMap=u0,u1,p2
  Prelookup : PreLookup  BreakpointsDataSource=Input port  BreakpointsData=[10:10:110]  ExtrapMethod=Linear
      settings: InputPortMap=u0,p1
  Selector : Selector  InputPortWidth=3  IndexOptions=Index vector (dialog)  Indices=1  OutputSizes=1
  Selector1 : Selector  InputPortWidth=3  IndexOptions=Index vector (dialog)  Indices=3  OutputSizes=1
  Selector10 : Selector  InputPortWidth=3  IndexOptions=Index vector (dialog)  Indices=2  OutputSizes=1
  Sum : Sum  Inputs=++|
  Sum1 : Sum  Inputs=|-+
  Sum2 : Sum  Inputs=|-+
  WaveVx1 : Outport
  WaveVy1 : Outport  Port=2
  wires:
  Cross Product/1 -> Selector/1, Selector10/1  "Rot"
  VxVec/1 -> Interpolation Using Prelookup/3
  Sum/1 -> Prelookup/1
  Prelookup/2 -> Interpolation Using Prelookup1/2, Interpolation Using Prelookup/2
  Zrot1/1 -> Selector1/1, Cross Product/2  "Zrot"
  Zplat/1 -> Sum/2
  Constant1/1 -> Prelookup/2
  Prelookup/1 -> Interpolation Using Prelookup1/1, Interpolation Using Prelookup/1
  Selector/1 -> Sum2/1
  Sum2/1 -> WaveVx1/1
  Selector10/1 -> Sum1/1
  Interpolation Using Prelookup/1 -> Sum2/2
  Interpolation Using Prelookup1/1 -> Sum1/2
  Hull rot spd/1 -> Cross Product/1
  Sum1/1 -> WaveVy1/1
  VyVec/1 -> Interpolation Using Prelookup1/3
  Selector1/1 -> Sum/1

== system SM_Offshore_Windturbine/HULL/Viscous loads/Subsystem1/Wave velocities/Subsystem1 ==
  Hull rot spd : Inport
  Zrot1 : Inport  Port=2
  Zplat : Inport  Port=3
  VxVec : Inport  Port=4
  VyVec : Inport  Port=5
  Constant1 : Constant  Value=par.wave.velocities.Z
  Cross Product : vrlib/Utilities/Cross Product
  Interpolation Using Prelookup : Interpolation_n-D  NumberOfTableDimensions=1  TableSource=Input port  InternalRulePriority=Speed
      settings: InputPortMap=u0,u1,p2
  Interpolation Using Prelookup1 : Interpolation_n-D  NumberOfTableDimensions=1  TableSource=Input port  InternalRulePriority=Speed
      settings: InputPortMap=u0,u1,p2
  Prelookup : PreLookup  BreakpointsDataSource=Input port  BreakpointsData=[10:10:110]  ExtrapMethod=Linear
      settings: InputPortMap=u0,p1
  Selector : Selector  InputPortWidth=3  IndexOptions=Index vector (dialog)  Indices=1  OutputSizes=1
  Selector1 : Selector  InputPortWidth=3  IndexOptions=Index vector (dialog)  Indices=3  OutputSizes=1
  Selector10 : Selector  InputPortWidth=3  IndexOptions=Index vector (dialog)  Indices=2  OutputSizes=1
  Sum : Sum  Inputs=++|
  Sum1 : Sum  Inputs=|-+
  Sum2 : Sum  Inputs=|-+
  WaveVx1 : Outport
  WaveVy1 : Outport  Port=2
  wires:
  Selector1/1 -> Sum/1
  VyVec/1 -> Interpolation Using Prelookup1/3
  Sum1/1 -> WaveVy1/1
  Hull rot spd/1 -> Cross Product/1
  Interpolation Using Prelookup1/1 -> Sum1/2
  Interpolation Using Prelookup/1 -> Sum2/2
  Selector10/1 -> Sum1/1
  Sum2/1 -> WaveVx1/1
  Selector/1 -> Sum2/1
  Prelookup/1 -> Interpolation Using Prelookup/1, Interpolation Using Prelookup1/1
  Constant1/1 -> Prelookup/2
  Zplat/1 -> Sum/2
  Zrot1/1 -> Cross Product/2, Selector1/1  "Zrot"
  Prelookup/2 -> Interpolation Using Prelookup/2, Interpolation Using Prelookup1/2
  Sum/1 -> Prelookup/1
  VxVec/1 -> Interpolation Using Prelookup/3
  Cross Product/1 -> Selector10/1, Selector/1  "Rot"

== system SM_Offshore_Windturbine/HULL/Viscous loads/Subsystem1/Wave velocities/Subsystem2 ==
  Hull rot spd : Inport
  Zrot1 : Inport  Port=2
  Zplat : Inport  Port=3
  VxVec : Inport  Port=4
  VyVec : Inport  Port=5
  Constant1 : Constant  Value=par.wave.velocities.Z
  Cross Product : vrlib/Utilities/Cross Product
  Interpolation Using Prelookup : Interpolation_n-D  NumberOfTableDimensions=1  TableSource=Input port  InternalRulePriority=Speed
      settings: InputPortMap=u0,u1,p2
  Interpolation Using Prelookup1 : Interpolation_n-D  NumberOfTableDimensions=1  TableSource=Input port  InternalRulePriority=Speed
      settings: InputPortMap=u0,u1,p2
  Prelookup : PreLookup  BreakpointsDataSource=Input port  BreakpointsData=[10:10:110]  ExtrapMethod=Linear
      settings: InputPortMap=u0,p1
  Selector : Selector  InputPortWidth=3  IndexOptions=Index vector (dialog)  Indices=1  OutputSizes=1
  Selector1 : Selector  InputPortWidth=3  IndexOptions=Index vector (dialog)  Indices=3  OutputSizes=1
  Selector10 : Selector  InputPortWidth=3  IndexOptions=Index vector (dialog)  Indices=2  OutputSizes=1
  Sum : Sum  Inputs=++|
  Sum1 : Sum  Inputs=|-+
  Sum2 : Sum  Inputs=|-+
  WaveVx1 : Outport
  WaveVy1 : Outport  Port=2
  wires:
  Cross Product/1 -> Selector/1, Selector10/1  "Rot"
  VxVec/1 -> Interpolation Using Prelookup/3
  Sum/1 -> Prelookup/1
  Prelookup/2 -> Interpolation Using Prelookup1/2, Interpolation Using Prelookup/2
  Zrot1/1 -> Selector1/1, Cross Product/2  "Zrot"
  Zplat/1 -> Sum/2
  Constant1/1 -> Prelookup/2
  Prelookup/1 -> Interpolation Using Prelookup1/1, Interpolation Using Prelookup/1
  Selector/1 -> Sum2/1
  Sum2/1 -> WaveVx1/1
  Selector10/1 -> Sum1/1
  Interpolation Using Prelookup/1 -> Sum2/2
  Interpolation Using Prelookup1/1 -> Sum1/2
  Hull rot spd/1 -> Cross Product/1
  Sum1/1 -> WaveVy1/1
  VyVec/1 -> Interpolation Using Prelookup1/3
  Selector1/1 -> Sum/1

== system SM_Offshore_Windturbine/HULL/Viscous loads/Subsystem1/Wave velocities/Subsystem3 ==
  Hull rot spd : Inport
  Zrot1 : Inport  Port=2
  Zplat : Inport  Port=3
  VxVec : Inport  Port=4
  VyVec : Inport  Port=5
  Constant1 : Constant  Value=par.wave.velocities.Z
  Cross Product : vrlib/Utilities/Cross Product
  Interpolation Using Prelookup : Interpolation_n-D  NumberOfTableDimensions=1  TableSource=Input port  InternalRulePriority=Speed
      settings: InputPortMap=u0,u1,p2
  Interpolation Using Prelookup1 : Interpolation_n-D  NumberOfTableDimensions=1  TableSource=Input port  InternalRulePriority=Speed
      settings: InputPortMap=u0,u1,p2
  Prelookup : PreLookup  BreakpointsDataSource=Input port  BreakpointsData=[10:10:110]  ExtrapMethod=Linear
      settings: InputPortMap=u0,p1
  Selector : Selector  InputPortWidth=3  IndexOptions=Index vector (dialog)  Indices=1  OutputSizes=1
  Selector1 : Selector  InputPortWidth=3  IndexOptions=Index vector (dialog)  Indices=3  OutputSizes=1
  Selector10 : Selector  InputPortWidth=3  IndexOptions=Index vector (dialog)  Indices=2  OutputSizes=1
  Sum : Sum  Inputs=++|
  Sum1 : Sum  Inputs=|-+
  Sum2 : Sum  Inputs=|-+
  WaveVx1 : Outport
  WaveVy1 : Outport  Port=2
  wires:
  Selector1/1 -> Sum/1
  VyVec/1 -> Interpolation Using Prelookup1/3
  Sum1/1 -> WaveVy1/1
  Hull rot spd/1 -> Cross Product/1
  Interpolation Using Prelookup1/1 -> Sum1/2
  Interpolation Using Prelookup/1 -> Sum2/2
  Selector10/1 -> Sum1/1
  Sum2/1 -> WaveVx1/1
  Selector/1 -> Sum2/1
  Prelookup/1 -> Interpolation Using Prelookup/1, Interpolation Using Prelookup1/1
  Constant1/1 -> Prelookup/2
  Zplat/1 -> Sum/2
  Zrot1/1 -> Cross Product/2, Selector1/1  "Zrot"
  Prelookup/2 -> Interpolation Using Prelookup/2, Interpolation Using Prelookup1/2
  Sum/1 -> Prelookup/1
  VxVec/1 -> Interpolation Using Prelookup/3
  Cross Product/1 -> Selector10/1, Selector/1  "Rot"

== system SM_Offshore_Windturbine/HULL/Viscous loads/Subsystem1/Wave velocities/Subsystem4 ==
  Hull rot spd : Inport
  Zrot1 : Inport  Port=2
  Zplat : Inport  Port=3
  VxVec : Inport  Port=4
  VyVec : Inport  Port=5
  Constant1 : Constant  Value=par.wave.velocities.Z
  Cross Product : vrlib/Utilities/Cross Product
  Interpolation Using Prelookup : Interpolation_n-D  NumberOfTableDimensions=1  TableSource=Input port  InternalRulePriority=Speed
      settings: InputPortMap=u0,u1,p2
  Interpolation Using Prelookup1 : Interpolation_n-D  NumberOfTableDimensions=1  TableSource=Input port  InternalRulePriority=Speed
      settings: InputPortMap=u0,u1,p2
  Prelookup : PreLookup  BreakpointsDataSource=Input port  BreakpointsData=[10:10:110]  ExtrapMethod=Linear
      settings: InputPortMap=u0,p1
  Selector : Selector  InputPortWidth=3  IndexOptions=Index vector (dialog)  Indices=1  OutputSizes=1
  Selector1 : Selector  InputPortWidth=3  IndexOptions=Index vector (dialog)  Indices=3  OutputSizes=1
  Selector10 : Selector  InputPortWidth=3  IndexOptions=Index vector (dialog)  Indices=2  OutputSizes=1
  Sum : Sum  Inputs=++|
  Sum1 : Sum  Inputs=|-+
  Sum2 : Sum  Inputs=|-+
  WaveVx1 : Outport
  WaveVy1 : Outport  Port=2
  wires:
  Cross Product/1 -> Selector/1, Selector10/1  "Rot"
  VxVec/1 -> Interpolation Using Prelookup/3
  Sum/1 -> Prelookup/1
  Prelookup/2 -> Interpolation Using Prelookup1/2, Interpolation Using Prelookup/2
  Zrot1/1 -> Selector1/1, Cross Product/2  "Zrot"
  Zplat/1 -> Sum/2
  Constant1/1 -> Prelookup/2
  Prelookup/1 -> Interpolation Using Prelookup1/1, Interpolation Using Prelookup/1
  Selector/1 -> Sum2/1
  Sum2/1 -> WaveVx1/1
  Selector10/1 -> Sum1/1
  Interpolation Using Prelookup/1 -> Sum2/2
  Interpolation Using Prelookup1/1 -> Sum1/2
  Hull rot spd/1 -> Cross Product/1
  Sum1/1 -> WaveVy1/1
  VyVec/1 -> Interpolation Using Prelookup1/3
  Selector1/1 -> Sum/1

== system SM_Offshore_Windturbine/HULL/Viscous loads/Subsystem1/Wave velocities/Subsystem5 ==
  Hull rot spd : Inport
  Zrot1 : Inport  Port=2
  Zplat : Inport  Port=3
  VxVec : Inport  Port=4
  VyVec : Inport  Port=5
  Constant1 : Constant  Value=par.wave.velocities.Z
  Cross Product : vrlib/Utilities/Cross Product
  Interpolation Using Prelookup : Interpolation_n-D  NumberOfTableDimensions=1  TableSource=Input port  InternalRulePriority=Speed
      settings: InputPortMap=u0,u1,p2
  Interpolation Using Prelookup1 : Interpolation_n-D  NumberOfTableDimensions=1  TableSource=Input port  InternalRulePriority=Speed
      settings: InputPortMap=u0,u1,p2
  Prelookup : PreLookup  BreakpointsDataSource=Input port  BreakpointsData=[10:10:110]  ExtrapMethod=Linear
      settings: InputPortMap=u0,p1
  Selector : Selector  InputPortWidth=3  IndexOptions=Index vector (dialog)  Indices=1  OutputSizes=1
  Selector1 : Selector  InputPortWidth=3  IndexOptions=Index vector (dialog)  Indices=3  OutputSizes=1
  Selector10 : Selector  InputPortWidth=3  IndexOptions=Index vector (dialog)  Indices=2  OutputSizes=1
  Sum : Sum  Inputs=++|
  Sum1 : Sum  Inputs=|-+
  Sum2 : Sum  Inputs=|-+
  WaveVx1 : Outport
  WaveVy1 : Outport  Port=2
  wires:
  Selector1/1 -> Sum/1
  VyVec/1 -> Interpolation Using Prelookup1/3
  Sum1/1 -> WaveVy1/1
  Hull rot spd/1 -> Cross Product/1
  Interpolation Using Prelookup1/1 -> Sum1/2
  Interpolation Using Prelookup/1 -> Sum2/2
  Selector10/1 -> Sum1/1
  Sum2/1 -> WaveVx1/1
  Selector/1 -> Sum2/1
  Prelookup/1 -> Interpolation Using Prelookup/1, Interpolation Using Prelookup1/1
  Constant1/1 -> Prelookup/2
  Zplat/1 -> Sum/2
  Zrot1/1 -> Cross Product/2, Selector1/1  "Zrot"
  Prelookup/2 -> Interpolation Using Prelookup/2, Interpolation Using Prelookup1/2
  Sum/1 -> Prelookup/1
  VxVec/1 -> Interpolation Using Prelookup/3
  Cross Product/1 -> Selector10/1, Selector/1  "Rot"

== system SM_Offshore_Windturbine/HULL/Viscous loads/Subsystem1/Wave velocities/Subsystem6 ==
  Hull rot spd : Inport
  Zrot1 : Inport  Port=2
  Zplat : Inport  Port=3
  VxVec : Inport  Port=4
  VyVec : Inport  Port=5
  Constant1 : Constant  Value=par.wave.velocities.Z
  Cross Product : vrlib/Utilities/Cross Product
  Interpolation Using Prelookup : Interpolation_n-D  NumberOfTableDimensions=1  TableSource=Input port  InternalRulePriority=Speed
      settings: InputPortMap=u0,u1,p2
  Interpolation Using Prelookup1 : Interpolation_n-D  NumberOfTableDimensions=1  TableSource=Input port  InternalRulePriority=Speed
      settings: InputPortMap=u0,u1,p2
  Prelookup : PreLookup  BreakpointsDataSource=Input port  BreakpointsData=[10:10:110]  ExtrapMethod=Linear
      settings: InputPortMap=u0,p1
  Selector : Selector  InputPortWidth=3  IndexOptions=Index vector (dialog)  Indices=1  OutputSizes=1
  Selector1 : Selector  InputPortWidth=3  IndexOptions=Index vector (dialog)  Indices=3  OutputSizes=1
  Selector10 : Selector  InputPortWidth=3  IndexOptions=Index vector (dialog)  Indices=2  OutputSizes=1
  Sum : Sum  Inputs=++|
  Sum1 : Sum  Inputs=|-+
  Sum2 : Sum  Inputs=|-+
  WaveVx1 : Outport
  WaveVy1 : Outport  Port=2
  wires:
  Cross Product/1 -> Selector/1, Selector10/1  "Rot"
  VxVec/1 -> Interpolation Using Prelookup/3
  Sum/1 -> Prelookup/1
  Prelookup/2 -> Interpolation Using Prelookup1/2, Interpolation Using Prelookup/2
  Zrot1/1 -> Selector1/1, Cross Product/2  "Zrot"
  Zplat/1 -> Sum/2
  Constant1/1 -> Prelookup/2
  Prelookup/1 -> Interpolation Using Prelookup1/1, Interpolation Using Prelookup/1
  Selector/1 -> Sum2/1
  Sum2/1 -> WaveVx1/1
  Selector10/1 -> Sum1/1
  Interpolation Using Prelookup/1 -> Sum2/2
  Interpolation Using Prelookup1/1 -> Sum1/2
  Hull rot spd/1 -> Cross Product/1
  Sum1/1 -> WaveVy1/1
  VyVec/1 -> Interpolation Using Prelookup1/3
  Selector1/1 -> Sum/1

== system SM_Offshore_Windturbine/HULL/Viscous loads/Subsystem1/Wave velocities/Subsystem7 ==
  Hull rot spd : Inport
  Zrot1 : Inport  Port=2
  Zplat : Inport  Port=3
  VxVec : Inport  Port=4
  VyVec : Inport  Port=5
  Constant1 : Constant  Value=par.wave.velocities.Z
  Cross Product : vrlib/Utilities/Cross Product
  Interpolation Using Prelookup : Interpolation_n-D  NumberOfTableDimensions=1  TableSource=Input port  InternalRulePriority=Speed
      settings: InputPortMap=u0,u1,p2
  Interpolation Using Prelookup1 : Interpolation_n-D  NumberOfTableDimensions=1  TableSource=Input port  InternalRulePriority=Speed
      settings: InputPortMap=u0,u1,p2
  Prelookup : PreLookup  BreakpointsDataSource=Input port  BreakpointsData=[10:10:110]  ExtrapMethod=Linear
      settings: InputPortMap=u0,p1
  Selector : Selector  InputPortWidth=3  IndexOptions=Index vector (dialog)  Indices=1  OutputSizes=1
  Selector1 : Selector  InputPortWidth=3  IndexOptions=Index vector (dialog)  Indices=3  OutputSizes=1
  Selector10 : Selector  InputPortWidth=3  IndexOptions=Index vector (dialog)  Indices=2  OutputSizes=1
  Sum : Sum  Inputs=++|
  Sum1 : Sum  Inputs=|-+
  Sum2 : Sum  Inputs=|-+
  WaveVx1 : Outport
  WaveVy1 : Outport  Port=2
  wires:
  Selector1/1 -> Sum/1
  VyVec/1 -> Interpolation Using Prelookup1/3
  Sum1/1 -> WaveVy1/1
  Hull rot spd/1 -> Cross Product/1
  Interpolation Using Prelookup1/1 -> Sum1/2
  Interpolation Using Prelookup/1 -> Sum2/2
  Selector10/1 -> Sum1/1
  Sum2/1 -> WaveVx1/1
  Selector/1 -> Sum2/1
  Prelookup/1 -> Interpolation Using Prelookup/1, Interpolation Using Prelookup1/1
  Constant1/1 -> Prelookup/2
  Zplat/1 -> Sum/2
  Zrot1/1 -> Cross Product/2, Selector1/1  "Zrot"
  Prelookup/2 -> Interpolation Using Prelookup/2, Interpolation Using Prelookup1/2
  Sum/1 -> Prelookup/1
  VxVec/1 -> Interpolation Using Prelookup/3
  Cross Product/1 -> Selector10/1, Selector/1  "Rot"

== system SM_Offshore_Windturbine/HULL/Viscous loads/Subsystem1/Wave velocities/Subsystem8 ==
  Hull rot spd : Inport
  Zrot1 : Inport  Port=2
  Zplat : Inport  Port=3
  VxVec : Inport  Port=4
  VyVec : Inport  Port=5
  Constant1 : Constant  Value=par.wave.velocities.Z
  Cross Product : vrlib/Utilities/Cross Product
  Interpolation Using Prelookup : Interpolation_n-D  NumberOfTableDimensions=1  TableSource=Input port  InternalRulePriority=Speed
      settings: InputPortMap=u0,u1,p2
  Interpolation Using Prelookup1 : Interpolation_n-D  NumberOfTableDimensions=1  TableSource=Input port  InternalRulePriority=Speed
      settings: InputPortMap=u0,u1,p2
  Prelookup : PreLookup  BreakpointsDataSource=Input port  BreakpointsData=[10:10:110]  ExtrapMethod=Linear
      settings: InputPortMap=u0,p1
  Selector : Selector  InputPortWidth=3  IndexOptions=Index vector (dialog)  Indices=1  OutputSizes=1
  Selector1 : Selector  InputPortWidth=3  IndexOptions=Index vector (dialog)  Indices=3  OutputSizes=1
  Selector10 : Selector  InputPortWidth=3  IndexOptions=Index vector (dialog)  Indices=2  OutputSizes=1
  Sum : Sum  Inputs=++|
  Sum1 : Sum  Inputs=|-+
  Sum2 : Sum  Inputs=|-+
  WaveVx1 : Outport
  WaveVy1 : Outport  Port=2
  wires:
  Cross Product/1 -> Selector/1, Selector10/1  "Rot"
  VxVec/1 -> Interpolation Using Prelookup/3
  Sum/1 -> Prelookup/1
  Prelookup/2 -> Interpolation Using Prelookup1/2, Interpolation Using Prelookup/2
  Zrot1/1 -> Selector1/1, Cross Product/2  "Zrot"
  Zplat/1 -> Sum/2
  Constant1/1 -> Prelookup/2
  Prelookup/1 -> Interpolation Using Prelookup1/1, Interpolation Using Prelookup/1
  Selector/1 -> Sum2/1
  Sum2/1 -> WaveVx1/1
  Selector10/1 -> Sum1/1
  Interpolation Using Prelookup/1 -> Sum2/2
  Interpolation Using Prelookup1/1 -> Sum1/2
  Hull rot spd/1 -> Cross Product/1
  Sum1/1 -> WaveVy1/1
  VyVec/1 -> Interpolation Using Prelookup1/3
  Selector1/1 -> Sum/1

== system SM_Offshore_Windturbine/HULL/Viscous loads/Subsystem1/Wave velocities/Subsystem9 ==
  Hull rot spd : Inport
  Zrot1 : Inport  Port=2
  Zplat : Inport  Port=3
  VxVec : Inport  Port=4
  VyVec : Inport  Port=5
  Constant1 : Constant  Value=par.wave.velocities.Z
  Cross Product : vrlib/Utilities/Cross Product
  Interpolation Using Prelookup : Interpolation_n-D  NumberOfTableDimensions=1  TableSource=Input port  InternalRulePriority=Speed
      settings: InputPortMap=u0,u1,p2
  Interpolation Using Prelookup1 : Interpolation_n-D  NumberOfTableDimensions=1  TableSource=Input port  InternalRulePriority=Speed
      settings: InputPortMap=u0,u1,p2
  Prelookup : PreLookup  BreakpointsDataSource=Input port  BreakpointsData=[10:10:110]  ExtrapMethod=Linear
      settings: InputPortMap=u0,p1
  Selector : Selector  InputPortWidth=3  IndexOptions=Index vector (dialog)  Indices=1  OutputSizes=1
  Selector1 : Selector  InputPortWidth=3  IndexOptions=Index vector (dialog)  Indices=3  OutputSizes=1
  Selector10 : Selector  InputPortWidth=3  IndexOptions=Index vector (dialog)  Indices=2  OutputSizes=1
  Sum : Sum  Inputs=++|
  Sum1 : Sum  Inputs=|-+
  Sum2 : Sum  Inputs=|-+
  WaveVx1 : Outport
  WaveVy1 : Outport  Port=2
  wires:
  Selector1/1 -> Sum/1
  VyVec/1 -> Interpolation Using Prelookup1/3
  Sum1/1 -> WaveVy1/1
  Hull rot spd/1 -> Cross Product/1
  Interpolation Using Prelookup1/1 -> Sum1/2
  Interpolation Using Prelookup/1 -> Sum2/2
  Selector10/1 -> Sum1/1
  Sum2/1 -> WaveVx1/1
  Selector/1 -> Sum2/1
  Prelookup/1 -> Interpolation Using Prelookup/1, Interpolation Using Prelookup1/1
  Constant1/1 -> Prelookup/2
  Zplat/1 -> Sum/2
  Zrot1/1 -> Cross Product/2, Selector1/1  "Zrot"
  Prelookup/2 -> Interpolation Using Prelookup/2, Interpolation Using Prelookup1/2
  Sum/1 -> Prelookup/1
  VxVec/1 -> Interpolation Using Prelookup/3
  Cross Product/1 -> Selector10/1, Selector/1  "Rot"
